simulink model "LPV_POWERSHARING"  (R2017b)
settings: Solver=ode1  StartTime=0.0  StopTime=30  FixedStep=2e-5  RelTol=1e-3  EnableMultiTasking=on
undefined symbols (not defined in the file or in its folder): aa, Acid, bb, cc, dd, Lead
libraries: powerlib x22, simulink x9, electricdrivelib x2
settings Model: Creator=MEHDI  LastModifiedBy=mac
settings SolverCC: ZeroCrossControl=DisableAll
settings DataIOCC: LimitDataPoints=on  SaveFormat=Array  SignalLoggingSaveFormat=ModelDataLogs
settings OptimizationCC: LifeSpan=inf
settings DebuggingCC: UnderspecifiedInitializationDetection=Classic  MergeDetectMultiDrivingBlocksExec=none  SolverPrmCheckMsg=warning  FcnCallInpInsideContextMsg=warning  StateNameClashWarn=warning  SFUnexpectedBacktrackingDiag=warning  SFNoUnconditionalDefaultTransitionDiag=warning  SFExecutionAtInitializationDiag=none
settings HardwareCC: ProdBitPerPointer=32  ProdBitPerSizeT=32  ProdBitPerPtrDiffT=32  ProdLargestAtomicFloat=None  ProdIntDivRoundTo=Undefined  ProdEndianess=Unspecified  ProdWordSize=32  ProdHWDeviceType=32-bit Generic
settings ModelReferenceCC: PropagateSignalLabelsOutOfModel=off
settings CodeAppCC: StateflowObjectComments=on
settings GRTTargetCC: TargetLangStandard=C89/C90 (ANSI)  GeneratePreprocessorConditionals=Disable all  CombineOutputUpdateFcns=off  GRTInterface=on
settings ConfigComp: CovMetricSettings=dw  CovHtmlReporting=on  CovSaveCumulativeToWorkspaceVar=on  CovSaveSingleToWorkspaceVar=on  CovExternalEMLEnable=off

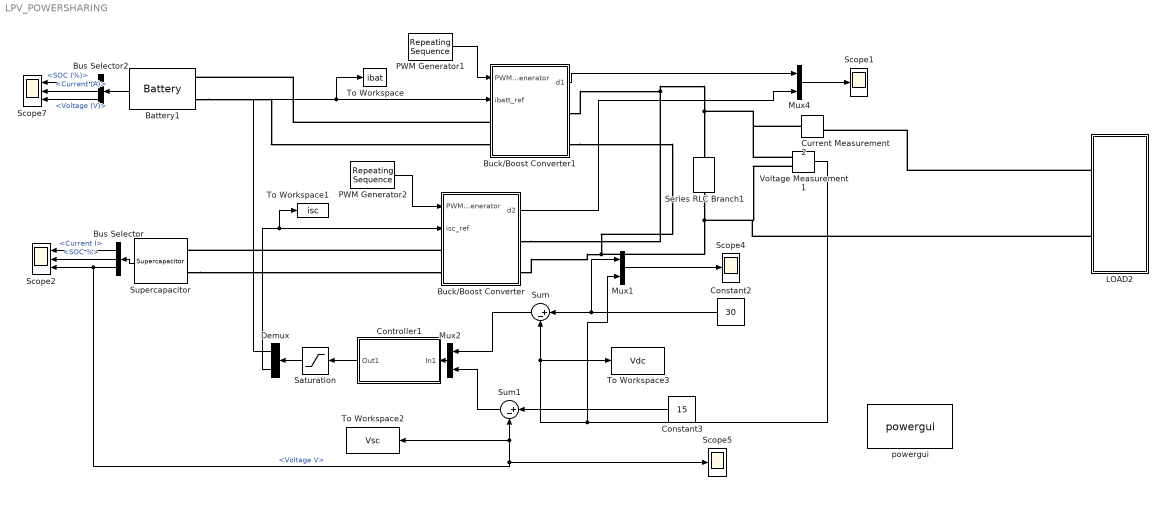
== system LPV_POWERSHARING ==
  Battery1 : electricdrivelib/Extra Sources/Battery  BatType=Lead-Acid  ShowTempParam=off  ThermalPreset=no  ShowAgeParam=off  NomV=12  NomQ=100  SOC=100  Batt_Tr=30  PresetModel=on  MaxQ=104.1667  MinV=9  FullV=13.0658  Dis_rate=20  R=0.0012  Normal_OP=31.0278  expZone="[12.2171     0.333333]"  current=[30 40]  Units=Time  Tci=20  NomT=20  T2=-30  MaxQ2=4.8  FullV2=7.1  Normal_OP2=5.655  expZone2="[6.58           1]"  Rca=0.6  ti=2000  Dp=0  Neq0=0  Tsim=1e6  Ta1=25  Qeol=5.4*0.9  Reol=0.013333*1.2  Char_age=[2.3478, 3]  Dis_age=[2.3478, 10]  N1=1500  N2=10500  N3=1000  N4=1400  Ta2=45  N5=950
  Buck/Boost Converter : Subsystem
  Buck/Boost Converter1 : Subsystem
  Bus Selector : BusSelector  OutputSignals=Current I,SOC %,Voltage V
  Bus Selector2 : BusSelector  OutputSignals=SOC (%),Current (A),Voltage (V)
  Constant2 : Constant  Value=30
  Constant3 : Constant  Value=15
  Controller1 : Subsystem  mask(H_infty CONTROLLER){ae=aa, be=bb, ce=cc, de=dd}
      mask prompts: ae "Controller Matrix A:"; be "Controller Matrix B:"; ce "Controller Matrix C:"; de "Controller Matrix D:"
      mask help:
      | H_infty controller.
      | (Requires Control Toolbox and RCT)
      mask Help: H_infty controller design. Mask and unmask this block to see how it works.
      mask Display: disp('H_infty Controller')
  Current Measurement2 : powerlib/Measurements/Current Measurement  PhasorSimulation=off  OutputType=Complex  PSBequivalent=0
  Demux : Demux  Outputs=2
  LOAD2 : Subsystem
  Mux1 : Mux  Inputs=2
  Mux2 : Mux  Inputs=2
  Mux4 : Mux  Inputs=2
  PWM Generator1 : simulink/Sources/Repeating Sequence  rep_seq_t=[0 1/10000]  rep_seq_y=[0 1]
  PWM Generator2 : simulink/Sources/Repeating Sequence  rep_seq_t=[0 1/10000]  rep_seq_y=[0 1]
  Saturation : Saturate  UpperLimit=6  LowerLimit=-6
  Scope1 : Scope
  Scope2 : Scope  NumInputPorts=3
  Scope4 : Scope
  Scope5 : Scope
  Scope7 : Scope  NumInputPorts=3
  Series RLC Branch1 : powerlib/Elements/Series RLC Branch  LConnTagsString=__new0  RConnTagsString=__new0  BranchType=C  Resistance=10  Inductance=1e-3  SetiL0=off  InitialCurrent=0  Capacitance=2200e-6  Setx0=off  InitialVoltage=0  Measurements=None
  Sum : Sum  Inputs=|+-
  Sum1 : Sum  Inputs=|+-
  Supercapacitor : electricdrivelib/Extra Sources/Supercapacitor  C=500  Rdc=2.1e-3  Voltage=16  Ns=6  Np=1  Vinit=14  Temp=25  PresetModel=on  EstParam=off  Nc=1  r=1e-9  epsilon=6.0208e-10  Ich=10  Vstern="[0.161  2.7  7.8]"  Self_dis=on  Ioc=10  Vself="[48  47.8  47.06  44.65]"  demandeplot=off  I=10.2  Units=sec  Vmax=17  If=5.2e-3  deltaV=0.3  alpha=0.3  sec=1988
      settings: SourceProductName=Simscape Power Systems  SourceProductBaseCode=PS
  To Workspace : ToWorkspace  VariableName=ibat  SampleTime=-1
  To Workspace1 : ToWorkspace  VariableName=isc  SampleTime=-1
  To Workspace2 : ToWorkspace  VariableName=Vsc  SampleTime=-1
  To Workspace3 : ToWorkspace  VariableName=Vdc  SampleTime=-1
  Voltage Measurement1 : powerlib/Measurements/Voltage Measurement  PhasorSimulation=off  OutputType=Complex  PSBequivalent=0
  powergui : powerlib/powergui  Priority=1  SimulationMode=Discrete  SampleTime=2e-5  frequency=60  Iterations=50  frequencyindice=0  Pbase=100e6  ErrMax=1e-4  UnitsV=kV  UnitsW=MW  buscounter=0  FunctionMessages=off  echomessages=off  EnableUseOfTLC=off  CurrentSourceSwitches=off  DisableSnubberDevices=off  DisableRonSwitches=off  DisableVfSwitches=off  DisplayEquations=off  SolverType=Tustin  Interpol=off  ExternalGateDelay=off  methode=off  Ts=0  x0status=blocks  SPID=off  SwTol=0  HookPort=off  RestoreLinks=warning  ResistiveCurrentMeasurement=off  Frange=[0:1:1000]  Ylog=on  Xlog=on  ShowGrid=on  save=on  variable=ZDa  structure=Data_bat  ZoomFFT=off  StartTime=0.0  cycles=1  DisplayStyle=1  fundamental=60  FreqAxis=off  MaxFrequency=1000  frequencyindicesteady=10  RmsSteady=1  display=off
  wires:
  PWM Generator2/1 -> Buck/Boost Converter/1(PWM Generator)
  Supercapacitor/1 -> Bus Selector/1
  Bus Selector/1 -> Scope2/1  "<Current I>"
  Bus Selector/2 -> Scope2/2  "<SOC %>"
  Bus Selector/3 -> To Workspace2/1, Sum1/2, Scope5/1, Scope2/3  "<Voltage V>"
  Voltage Measurement1/1 -> Mux1/2, To Workspace3/1, Sum/2
  Mux1/1 -> Scope4/1
  Constant2/1 -> Mux1/1, Sum/1
  Mux2/1 -> Controller1/1(In1)
  Constant3/1 -> Sum1/1
  PWM Generator1/1 -> Buck/Boost Converter1/1(PWM Generator)
  Battery1/1 -> Bus Selector2/1
  Bus Selector2/1 -> Scope7/1  "<SOC (%)>"
  Bus Selector2/2 -> Scope7/2  "<Current (A)>"
  Bus Selector2/3 -> Scope7/3  "<Voltage (V)>"
  Mux4/1 -> Scope1/1
  Buck/Boost Converter1/1(d1) -> Mux4/1
  Buck/Boost Converter/1(d2) -> Mux4/2
  Controller1/1(Out1) -> Saturation/1
  Saturation/1 -> Demux/1
  Sum/1 -> Mux2/1
  Sum1/1 -> Mux2/2
  Demux/1 -> To Workspace/1, Buck/Boost Converter1/2(ibatt_ref)
  Demux/2 -> To Workspace1/1, Buck/Boost Converter/2(isc_ref)
  connections:
  Buck/Boost Converter/RConn1 -- Current Measurement2/LConn1 -- Voltage Measurement1/LConn1 -- Series RLC Branch1/RConn1 -- Buck/Boost Converter1/RConn1
  LOAD2/LConn2 -- Voltage Measurement1/LConn2 -- Series RLC Branch1/LConn1 -- Buck/Boost Converter1/RConn2 -- Buck/Boost Converter/RConn2
  Buck/Boost Converter1/LConn1 -- Battery1/LConn1
  Buck/Boost Converter/LConn1 -- Supercapacitor/LConn1
  Battery1/LConn2 -- Buck/Boost Converter1/LConn2
  Supercapacitor/LConn2 -- Buck/Boost Converter/LConn2
  LOAD2/LConn1 -- Current Measurement2/RConn1

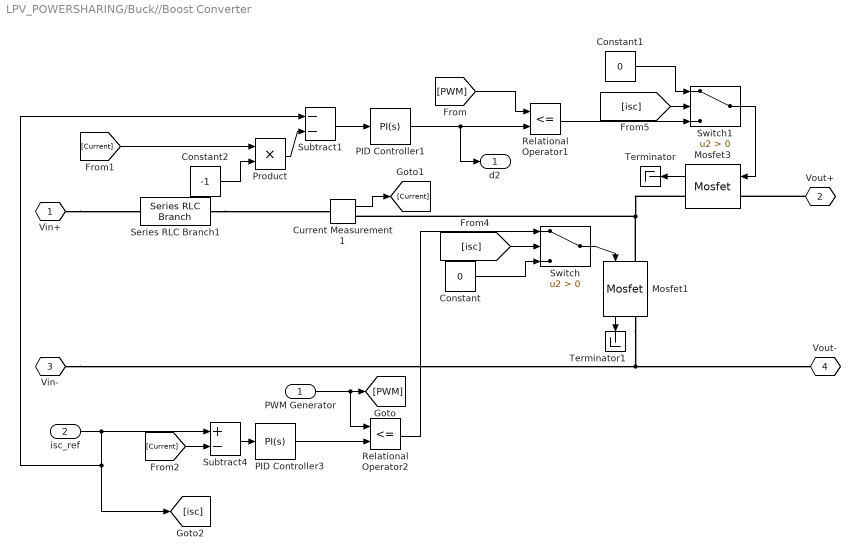
== system LPV_POWERSHARING/Buck//Boost Converter ==
  PWM Generator : Inport
  isc_ref : Inport  Port=2
  Constant : Constant  Value=0
  Constant1 : Constant  Value=0
  Constant2 : Constant  Value=-1
  Current Measurement1 : powerlib/Measurements/Current Measurement  PhasorSimulation=off  OutputType=Complex  PSBequivalent=0
  Mosfet1 : powerlib/Power Electronics/Mosfet  Ron=0.1  Lon=0  Rd=0.01  Vfd=0  IC=0  Rs=1e5  Cs=inf  Measurements=on
  Mosfet3 : powerlib/Power Electronics/Mosfet  Ron=0.1  Lon=0  Rd=0.01  Vfd=0  IC=0  Rs=1e5  Cs=inf  Measurements=on
  PID Controller1 : simulink/Continuous/PID Controller  Controller=PI  TimeDomain=Continuous-time  SampleTime=-1  IntegratorMethod=Forward Euler  FilterMethod=Forward Euler  Form=Ideal  UseFilter=on  ControllerParametersSource=internal  P=0.05  I=50  D=0  N=100  InitialConditionSource=internal  InitialConditionForIntegrator=0  InitialConditionForFilter=0  ExternalReset=none  LimitOutput=off  UpperSaturationLimit=1  LowerSaturationLimit=0  LinearizeAsGain=off  AntiWindupMode=none  Kb=1  TrackingMode=off  Kt=1  PParamMin=[]  PParamMax=[]  IParamMin=[]  IParamMax=[]  DParamMin=[]  DParamMax=[]  NParamMin=[]  NParamMax=[]  KbParamMin=[]  KbParamMax=[]  KtParamMin=[]  KtParamMax=[]  POutMin=[]  POutMax=[]  IOutMin=[]  IOutMax=[]  DOutMin=[]  DOutMax=[]  NOutMin=[]  NOutMax=[]  KbOutMin=[]  KbOutMax=[]  KtOutMin=[]  KtOutMax=[]  IntegratorOutMin=[]  IntegratorOutMax=[]  FilterOutMin=[]  FilterOutMax=[]  SumOutMin=[]  SumOutMax=[]  SumI1OutMin=[]  SumI1OutMax=[]  SumI2OutMin=[]  SumI2OutMax=[]  SumI3OutMin=[]  SumI3OutMax=[]  SumDOutMin=[]  SumDOutMax=[]  SaturationOutMin=[]  SaturationOutMax=[]  IntegratorContinuousStateAttributes=''  IntegratorStateMustResolveToSignalObject=off  IntegratorRTWStateStorageClass=Auto  FilterContinuousStateAttributes=''  FilterStateMustResolveToSignalObject=off  FilterRTWStateStorageClass=Auto  DifferentiatorICPrevScaledInput=0  DifferentiatorOutMin=[]  DifferentiatorOutMax=[]  InitialConditionSetting=State (most efficient)  FilterDiffOutCoefMin=[]  FilterDiffOutCoefMax=[]  SumDenOutMin=[]  SumDenOutMax=[]  SumNumOutMin=[]  SumNumOutMax=[]  ReciprocalOutMin=[]  ReciprocalOutMax=[]  DivideOutMin=[]  DivideOutMax=[]  TunerSelectOption=Transfer Function Based (PID Tuner App)
  PID Controller3 : simulink/Continuous/PID Controller  Controller=PI  TimeDomain=Continuous-time  SampleTime=-1  IntegratorMethod=Forward Euler  FilterMethod=Forward Euler  Form=Ideal  UseFilter=on  ControllerParametersSource=internal  P=0.05  I=50  D=0  N=100  InitialConditionSource=internal  InitialConditionForIntegrator=0  InitialConditionForFilter=0  ExternalReset=none  LimitOutput=off  UpperSaturationLimit=1  LowerSaturationLimit=0  LinearizeAsGain=off  AntiWindupMode=none  Kb=1  TrackingMode=off  Kt=1  PParamMin=[]  PParamMax=[]  IParamMin=[]  IParamMax=[]  DParamMin=[]  DParamMax=[]  NParamMin=[]  NParamMax=[]  KbParamMin=[]  KbParamMax=[]  KtParamMin=[]  KtParamMax=[]  POutMin=[]  POutMax=[]  IOutMin=[]  IOutMax=[]  DOutMin=[]  DOutMax=[]  NOutMin=[]  NOutMax=[]  KbOutMin=[]  KbOutMax=[]  KtOutMin=[]  KtOutMax=[]  IntegratorOutMin=[]  IntegratorOutMax=[]  FilterOutMin=[]  FilterOutMax=[]  SumOutMin=[]  SumOutMax=[]  SumI1OutMin=[]  SumI1OutMax=[]  SumI2OutMin=[]  SumI2OutMax=[]  SumI3OutMin=[]  SumI3OutMax=[]  SumDOutMin=[]  SumDOutMax=[]  SaturationOutMin=[]  SaturationOutMax=[]  IntegratorContinuousStateAttributes=''  IntegratorStateMustResolveToSignalObject=off  IntegratorRTWStateStorageClass=Auto  FilterContinuousStateAttributes=''  FilterStateMustResolveToSignalObject=off  FilterRTWStateStorageClass=Auto  DifferentiatorICPrevScaledInput=0  DifferentiatorOutMin=[]  DifferentiatorOutMax=[]  InitialConditionSetting=State (most efficient)  FilterDiffOutCoefMin=[]  FilterDiffOutCoefMax=[]  SumDenOutMin=[]  SumDenOutMax=[]  SumNumOutMin=[]  SumNumOutMax=[]  ReciprocalOutMin=[]  ReciprocalOutMax=[]  DivideOutMin=[]  DivideOutMax=[]  TunerSelectOption=Transfer Function Based (PID Tuner App)
  Product : Product  RndMeth=Zero
  Relational Operator1 : RelationalOperator  Operator=<=  OutDataTypeStr=boolean  RndMeth=Nearest
  Relational Operator2 : RelationalOperator  Operator=<=  OutDataTypeStr=boolean  RndMeth=Nearest
  Series RLC Branch1 : powerlib/Elements/Series RLC Branch  LConnTagsString=__new0  RConnTagsString=__new0  BranchType=L  Resistance=1  Inductance=1e-3  SetiL0=off  InitialCurrent=0  Capacitance=1e-6  Setx0=off  InitialVoltage=0  Measurements=None
  Subtract1 : Sum  Inputs=--
  Subtract4 : Sum  Inputs=+-
  Switch : Switch  Criteria=u2 > Threshold
  Switch1 : Switch  Criteria=u2 > Threshold
  Terminator : Terminator
  Terminator1 : Terminator
  Vin+ : PMIOPort  Tag=PMCPort  Port=1  Side=Left
  Vout+ : PMIOPort  Tag=PMCPort  Port=2  Side=Right
  Vin- : PMIOPort  Tag=PMCPort  Port=3  Side=Left
  Vout- : PMIOPort  Tag=PMCPort  Port=4  Side=Right
  d2 : Outport
  wires:
  PID Controller3/1 -> Relational Operator2/2
  Subtract4/1 -> PID Controller3/1
  PWM Generator/1 -> Relational Operator2/1, [PWM]
  isc_ref/1 -> [isc], Subtract1/1, Subtract4/1
  Switch/1 -> Mosfet1/1
  PID Controller1/1 -> d2/1, Relational Operator1/2
  Subtract1/1 -> PID Controller1/1
  [PWM] -> Relational Operator1/1
  [Current] -> Subtract4/2
  Product/1 -> Subtract1/2
  Constant2/1 -> Product/2
  Switch1/1 -> Mosfet3/1
  Relational Operator2/1 -> Switch/1
  Constant/1 -> Switch/3
  Constant1/1 -> Switch1/1
  Mosfet3/1 -> Terminator/1
  Mosfet1/1 -> Terminator1/1
  Relational Operator1/1 -> Switch1/3
  [isc] -> Switch/2
  [isc] -> Switch1/2
  Current Measurement1/1 -> [Current]
  [Current] -> Product/1
  connections:
  Vin-/RConn1 -- Vout-/RConn1 -- Mosfet1/RConn1
  Vin+/RConn1 -- Series RLC Branch1/LConn1
  Mosfet1/LConn1 -- Current Measurement1/RConn1 -- Mosfet3/RConn1
  Series RLC Branch1/RConn1 -- Current Measurement1/LConn1
  Vout+/RConn1 -- Mosfet3/LConn1

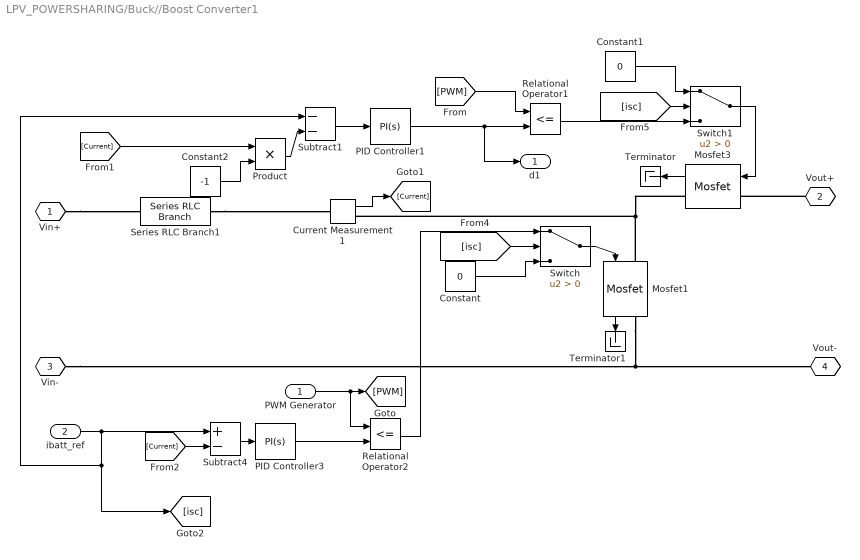
== system LPV_POWERSHARING/Buck//Boost Converter1 ==
  PWM Generator : Inport
  ibatt_ref : Inport  Port=2
  Constant : Constant  Value=0
  Constant1 : Constant  Value=0
  Constant2 : Constant  Value=-1
  Current Measurement1 : powerlib/Measurements/Current Measurement  PhasorSimulation=off  OutputType=Complex  PSBequivalent=0
  Mosfet1 : powerlib/Power Electronics/Mosfet  Ron=0.1  Lon=0  Rd=0.01  Vfd=0  IC=0  Rs=1e5  Cs=inf  Measurements=on
  Mosfet3 : powerlib/Power Electronics/Mosfet  Ron=0.1  Lon=0  Rd=0.01  Vfd=0  IC=0  Rs=1e5  Cs=inf  Measurements=on
  PID Controller1 : simulink/Continuous/PID Controller  Controller=PI  TimeDomain=Continuous-time  SampleTime=-1  IntegratorMethod=Forward Euler  FilterMethod=Forward Euler  Form=Ideal  UseFilter=on  ControllerParametersSource=internal  P=0.05  I=50  D=0  N=100  InitialConditionSource=internal  InitialConditionForIntegrator=0  InitialConditionForFilter=0  ExternalReset=none  LimitOutput=off  UpperSaturationLimit=1  LowerSaturationLimit=0  LinearizeAsGain=off  AntiWindupMode=none  Kb=1  TrackingMode=off  Kt=1  PParamMin=[]  PParamMax=[]  IParamMin=[]  IParamMax=[]  DParamMin=[]  DParamMax=[]  NParamMin=[]  NParamMax=[]  KbParamMin=[]  KbParamMax=[]  KtParamMin=[]  KtParamMax=[]  POutMin=[]  POutMax=[]  IOutMin=[]  IOutMax=[]  DOutMin=[]  DOutMax=[]  NOutMin=[]  NOutMax=[]  KbOutMin=[]  KbOutMax=[]  KtOutMin=[]  KtOutMax=[]  IntegratorOutMin=[]  IntegratorOutMax=[]  FilterOutMin=[]  FilterOutMax=[]  SumOutMin=[]  SumOutMax=[]  SumI1OutMin=[]  SumI1OutMax=[]  SumI2OutMin=[]  SumI2OutMax=[]  SumI3OutMin=[]  SumI3OutMax=[]  SumDOutMin=[]  SumDOutMax=[]  SaturationOutMin=[]  SaturationOutMax=[]  IntegratorContinuousStateAttributes=''  IntegratorStateMustResolveToSignalObject=off  IntegratorRTWStateStorageClass=Auto  FilterContinuousStateAttributes=''  FilterStateMustResolveToSignalObject=off  FilterRTWStateStorageClass=Auto  DifferentiatorICPrevScaledInput=0  DifferentiatorOutMin=[]  DifferentiatorOutMax=[]  InitialConditionSetting=State (most efficient)  FilterDiffOutCoefMin=[]  FilterDiffOutCoefMax=[]  SumDenOutMin=[]  SumDenOutMax=[]  SumNumOutMin=[]  SumNumOutMax=[]  ReciprocalOutMin=[]  ReciprocalOutMax=[]  DivideOutMin=[]  DivideOutMax=[]  TunerSelectOption=Transfer Function Based (PID Tuner App)
  PID Controller3 : simulink/Continuous/PID Controller  Controller=PI  TimeDomain=Continuous-time  SampleTime=-1  IntegratorMethod=Forward Euler  FilterMethod=Forward Euler  Form=Ideal  UseFilter=on  ControllerParametersSource=internal  P=0.05  I=50  D=0  N=100  InitialConditionSource=internal  InitialConditionForIntegrator=0  InitialConditionForFilter=0  ExternalReset=none  LimitOutput=off  UpperSaturationLimit=1  LowerSaturationLimit=0  LinearizeAsGain=off  AntiWindupMode=none  Kb=1  TrackingMode=off  Kt=1  PParamMin=[]  PParamMax=[]  IParamMin=[]  IParamMax=[]  DParamMin=[]  DParamMax=[]  NParamMin=[]  NParamMax=[]  KbParamMin=[]  KbParamMax=[]  KtParamMin=[]  KtParamMax=[]  POutMin=[]  POutMax=[]  IOutMin=[]  IOutMax=[]  DOutMin=[]  DOutMax=[]  NOutMin=[]  NOutMax=[]  KbOutMin=[]  KbOutMax=[]  KtOutMin=[]  KtOutMax=[]  IntegratorOutMin=[]  IntegratorOutMax=[]  FilterOutMin=[]  FilterOutMax=[]  SumOutMin=[]  SumOutMax=[]  SumI1OutMin=[]  SumI1OutMax=[]  SumI2OutMin=[]  SumI2OutMax=[]  SumI3OutMin=[]  SumI3OutMax=[]  SumDOutMin=[]  SumDOutMax=[]  SaturationOutMin=[]  SaturationOutMax=[]  IntegratorContinuousStateAttributes=''  IntegratorStateMustResolveToSignalObject=off  IntegratorRTWStateStorageClass=Auto  FilterContinuousStateAttributes=''  FilterStateMustResolveToSignalObject=off  FilterRTWStateStorageClass=Auto  DifferentiatorICPrevScaledInput=0  DifferentiatorOutMin=[]  DifferentiatorOutMax=[]  InitialConditionSetting=State (most efficient)  FilterDiffOutCoefMin=[]  FilterDiffOutCoefMax=[]  SumDenOutMin=[]  SumDenOutMax=[]  SumNumOutMin=[]  SumNumOutMax=[]  ReciprocalOutMin=[]  ReciprocalOutMax=[]  DivideOutMin=[]  DivideOutMax=[]  TunerSelectOption=Transfer Function Based (PID Tuner App)
  Product : Product  RndMeth=Zero
  Relational Operator1 : RelationalOperator  Operator=<=  OutDataTypeStr=boolean  RndMeth=Nearest
  Relational Operator2 : RelationalOperator  Operator=<=  OutDataTypeStr=boolean  RndMeth=Nearest
  Series RLC Branch1 : powerlib/Elements/Series RLC Branch  LConnTagsString=__new0  RConnTagsString=__new0  BranchType=L  Resistance=1  Inductance=1e-3  SetiL0=off  InitialCurrent=0  Capacitance=1e-6  Setx0=off  InitialVoltage=0  Measurements=None
  Subtract1 : Sum  Inputs=--
  Subtract4 : Sum  Inputs=+-
  Switch : Switch  Criteria=u2 > Threshold
  Switch1 : Switch  Criteria=u2 > Threshold
  Terminator : Terminator
  Terminator1 : Terminator
  Vin+ : PMIOPort  Tag=PMCPort  Port=1  Side=Left
  Vout+ : PMIOPort  Tag=PMCPort  Port=2  Side=Right
  Vin- : PMIOPort  Tag=PMCPort  Port=3  Side=Left
  Vout- : PMIOPort  Tag=PMCPort  Port=4  Side=Right
  d1 : Outport
  wires:
  [Current] -> Product/1
  Current Measurement1/1 -> [Current]
  [isc] -> Switch1/2
  [isc] -> Switch/2
  Relational Operator1/1 -> Switch1/3
  Mosfet1/1 -> Terminator1/1
  Mosfet3/1 -> Terminator/1
  Constant1/1 -> Switch1/1
  Constant/1 -> Switch/3
  Relational Operator2/1 -> Switch/1
  Switch1/1 -> Mosfet3/1
  Constant2/1 -> Product/2
  Product/1 -> Subtract1/2
  [Current] -> Subtract4/2
  [PWM] -> Relational Operator1/1
  Subtract1/1 -> PID Controller1/1
  PID Controller1/1 -> d1/1, Relational Operator1/2
  Switch/1 -> Mosfet1/1
  ibatt_ref/1 -> Subtract4/1, Subtract1/1, [isc]
  PWM Generator/1 -> [PWM], Relational Operator2/1
  Subtract4/1 -> PID Controller3/1
  PID Controller3/1 -> Relational Operator2/2
  connections:
  Vout+/RConn1 -- Mosfet3/LConn1
  Series RLC Branch1/RConn1 -- Current Measurement1/LConn1
  Mosfet3/RConn1 -- Current Measurement1/RConn1 -- Mosfet1/LConn1
  Vin+/RConn1 -- Series RLC Branch1/LConn1
  Mosfet1/RConn1 -- Vout-/RConn1 -- Vin-/RConn1

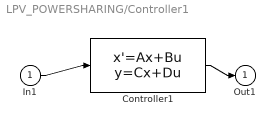
== system LPV_POWERSHARING/Controller1 ==
  In1 : Inport
  Controller1 : StateSpace  A=ae  B=be  C=ce  D=de  InitialCondition=0
  Out1 : Outport  InitialOutput=0
  wires:
  Controller1/1 -> Out1/1
  In1/1 -> Controller1/1

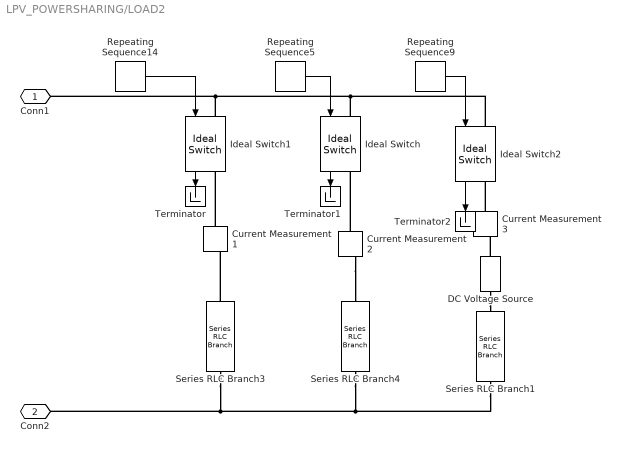
== system LPV_POWERSHARING/LOAD2 ==
  Current Measurement1 : powerlib/Measurements/Current Measurement  PhasorSimulation=off  OutputType=Complex  PSBequivalent=0
  Current Measurement2 : powerlib/Measurements/Current Measurement  PhasorSimulation=off  OutputType=Complex  PSBequivalent=0
  Current Measurement3 : powerlib/Measurements/Current Measurement  PhasorSimulation=off  OutputType=Complex  PSBequivalent=0
  DC Voltage Source : powerlib/Electrical Sources/DC Voltage Source  Amplitude=40  Measurements=None
  Ideal Switch : powerlib/Power Electronics/Ideal Switch  Ron=0.001  Lon=0  IC=0  Rs=1e5  Cs=inf  Measurements=on
  Ideal Switch1 : powerlib/Power Electronics/Ideal Switch  Ron=0.001  Lon=0  IC=0  Rs=1e5  Cs=inf  Measurements=on
  Ideal Switch2 : powerlib/Power Electronics/Ideal Switch  Ron=0.001  Lon=0  IC=0  Rs=1e5  Cs=inf  Measurements=on
  Repeating Sequence14 : simulink/Sources/Repeating Sequence  rep_seq_t=[0 1 2 2.0001 3 4 5 6]  rep_seq_y=[1 1 1 0 0 0 0 0]
  Repeating Sequence5 : simulink/Sources/Repeating Sequence  rep_seq_t="[0 1 2 2.0001 3  4 4.0001 5 6]"  rep_seq_y=[0 0 0 1 1 1 0 0 0]
  Repeating Sequence9 : simulink/Sources/Repeating Sequence  rep_seq_t="[0 1 2 3  4 4.0001 5 6]"  rep_seq_y="[0 0 0 0  0 1 1 1]"
  Series RLC Branch1 : powerlib/Elements/Series RLC Branch  LConnTagsString=__new0  RConnTagsString=__new0  BranchType=R  Resistance=10  Inductance=300e-3  SetiL0=off  InitialCurrent=0  Capacitance=2200e-6  Setx0=off  InitialVoltage=0  Measurements=None
  Series RLC Branch3 : powerlib/Elements/Series RLC Branch  LConnTagsString=__new0  RConnTagsString=__new0  BranchType=R  Resistance=30  Inductance=300e-3  SetiL0=off  InitialCurrent=0  Capacitance=2200e-6  Setx0=off  InitialVoltage=0  Measurements=None
  Series RLC Branch4 : powerlib/Elements/Series RLC Branch  LConnTagsString=__new0  RConnTagsString=__new0  BranchType=R  Resistance=15  Inductance=300e-3  SetiL0=off  InitialCurrent=0  Capacitance=2200e-6  Setx0=off  InitialVoltage=0  Measurements=None
  Terminator : Terminator
  Terminator1 : Terminator
  Terminator2 : Terminator
  Conn1 : PMIOPort  Port=1  Side=Left
  Conn2 : PMIOPort  Port=2  Side=Left
  wires:
  Repeating Sequence9/1 -> Ideal Switch2/1
  Repeating Sequence5/1 -> Ideal Switch/1
  Ideal Switch/1 -> Terminator1/1
  Ideal Switch1/1 -> Terminator/1
  Ideal Switch2/1 -> Terminator2/1
  Repeating Sequence14/1 -> Ideal Switch1/1
  connections:
  Ideal Switch/LConn1 -- Ideal Switch2/LConn1 -- Ideal Switch1/LConn1 -- Conn1/RConn1
  Current Measurement3/LConn1 -- Ideal Switch2/RConn1
  Current Measurement2/RConn1 -- Series RLC Branch4/RConn1
  Current Measurement2/LConn1 -- Ideal Switch/RConn1
  Series RLC Branch3/RConn1 -- Current Measurement1/RConn1
  Current Measurement1/LConn1 -- Ideal Switch1/RConn1
  Series RLC Branch4/LConn1 -- Series RLC Branch3/LConn1 -- Conn2/RConn1 -- Series RLC Branch1/LConn1
  DC Voltage Source/RConn1 -- Current Measurement3/RConn1
  DC Voltage Source/LConn1 -- Series RLC Branch1/RConn1
